simulink library "vmc"  (R2021b)
settings: Solver=VariableStepAuto  StartTime=0.0  StopTime=10.0  RelTol=1e-3
undefined symbols (not defined in the file or in its folder): AVMC_ACCDeltaTqIGain_X_kph, AVMC_ACCDeltaTqIGain_Y_mps2, AVMC_ACCDeltaTqPGain_X_kph, AVMC_ACCDeltaTqPGain_Y_kph, AVMC_ACCLongSteadyCtrl_X_kph, AVMC_AggressJerkPCT4AT_X_kph, AVMC_AggressJerkPCT_X_kph, AVMC_AggressLimitPCT4AT_X_kph, AVMC_AggressLimitPCT_X_kph, AVMC_CCLongSteadyCtrl_X_kph, AVMC_DISCDeltaTqIGain_X_kph, AVMC_DISCDeltaTqIGain_Y_mps2, AVMC_DISCDeltaTqPGain_X_kph, AVMC_DISCDeltaTqPGain_Y_kph, AVMC_DISCTrunAccJerk_X_s, AVMC_DISCTrunAccLimit_X_s, AVMC_ESCRegenOut_X_kph, AVMC_ESCRegenOut_Y_Deg, AVMC_ESCRegenOutEnSpd_X_Deg, AVMC_ISOAccLimit_X_mps, AVMC_ISODecLimit_X_mps, AVMC_ISOJerk_X_mps, AVMC_LatESCRegenOut_X_kph, AVMC_LatESCRegenOut_Y_Deg, AVMC_LongAccDeadZone_X_kph, AVMC_LongAccFiltTsforP2_X_Gps, AVMC_MCPresBaseTq_X_bar, AVMC_MSALongSteadyCtrl_X_kph, AVMC_MSAPedalOvrd2_X_kph, AVMC_MSAPedalOvrd_X_kph, AVMC_MSASpdBand_X_kph, AVMC_MSATqDownEndTq_X_kph, AVMC_MSATqDownTime_X_kph, AVMC_OPDDisSlideRate_X_Deg, AVMC_RDCDetectTime_X_kph, AVMC_RDCDetectTime_Y_pct, AVMC_RDCEnSlideRate_X_Deg, AVMC_RearWhlTqRatio_X_Nm, AVMC_RearWhlTqRatio_Y_gps, AVMC_RearWhlTqSlipGain_X_rat, AVMC_RearWhlTqSlipGain_Y_kph, AVMC_RearWhlTqSTRGGain_X_deg, AVMC_RearWhlTqSTRGGain_Y_kph, AVMC_RWSRrTSA2RWSPos_X_deg, AVMC_RWSSAS2FrtTSA_X_deg, AVMC_RWSVehSPD2RWSCoef_X_kph, AVMC_SoftJerkPCT_X_kph, AVMC_SoftLimitPCT_X_kph, AVMC_StESCYaw_X_kph, AVMC_StESCYaw_Y_Deg, AVMC_StESCYawCom_X_kph, AVMC_StESCYawCom_Y_Gps, AVMC_TMSpdBaseTq_X_rpm, AVMC_VehHoldBDecMap_X_kph, AVMC_VehHoldDecCtrlTime_X_kph, AVMC_VehHoldMCPPass_X_deg, C_TASK_10MS_S, C_TASK_5MS_S, DEG2RAD, ENUM_ACCAVAIL_AVAILABLE ... (+409)
libraries: hcu_lib x74, simulink x68, simulink_extras x3, $bdroot x2
(part 7 of 15)

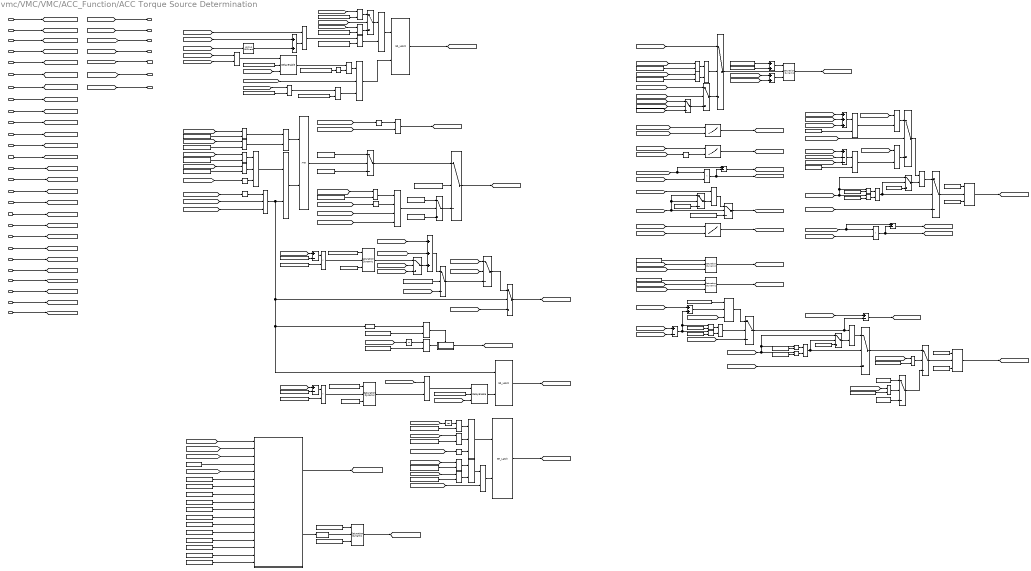
== system vmc/VMC/VMC/ACC_Function/ACC Torque Source Determination ==
  note: TRUE
  VTQD_DriverWhlTqDem_Nm : Inport
  VVMC_ADASWhlTqCal_Nm : Inport  Port=2
  VVMC_FeatArbitrFinal_enum : Inport  Port=3
  VTQD_LowIdleAccPedal_flg : Inport  Port=4
  VINP_ACCObjDist_m : Inport  Port=5
  VINP_TimeGapLevel_enum : Inport  Port=6
  VVMC_FeatArbitrSta_enum : Inport  Port=7
  VTQD_RegenMode_enum : Inport  Port=8
  VVMC_ADASActive_flg : Inport  Port=9
  task_time_s : Inport  Port=10
  VINP_LongAccel_Gps : Inport  Port=11
  VINP_VehSpeed_kph : Inport  Port=12
  VVMC_FrRrSlipSpd_kph : Inport  Port=13
  VVMC_CruzWhlTqReq_Nm : Inport  Port=14
  VVMC_CruzActive_flg : Inport  Port=15
  VVMC_MSAWhlTqReq_Nm : Inport  Port=16
  VVMC_MSAActive_flg : Inport  Port=17
  VTQD_RrEDUAvailBrkRgnTq_Nm : Inport  Port=18
  VTQD_FrEDUAvailBrkRgnTq_Nm : Inport  Port=19
  VPMM_DrivetrainSelect_enum : Inport  Port=20
  VINP_ACCObjRelSpd_mps : Inport  Port=21
  VINP_SASAngle_Deg : Inport  Port=22
  VDHP_ActAPSPosn_pct : Inport  Port=23
  VTQD_CreepBaseTqD_Nm : Inport  Port=24
  VVMC_ACCVehHoldReq_flg : Inport  Port=25
  VVMC_LongAcc_Gps : Inport  Port=26
  VVMC_ADASACCSta_enum : Inport  Port=27
  AND{,5..6,8..9,12} (6 alike) : Logic  AllPortsSameDT=off  OutDataTypeStr=boolean
  AND1 : Logic  Inputs=4  AllPortsSameDT=off  OutDataTypeStr=boolean
  AND11 : Logic  Inputs=3  AllPortsSameDT=off  OutDataTypeStr=boolean
  AND{2..4,7,13} (5 alike) : Logic  Operator=OR  AllPortsSameDT=off  OutDataTypeStr=boolean
  Abs : Abs
  Add{,9..11} (4 alike) : Sum
  Add{1,4..6,8,13} (6 alike) : Sum  Inputs=+-
  Add2 : Sum  Inputs=+++
  Add3 : Sum  Inputs=+--
  Add7 : Sum  Inputs=+++
  Cast To Single : DataTypeConversion  OutDataTypeStr=single
  Constant : Constant  Value=KVMC_ACCPedalOvrdSWC_flg
  Constant1 : Constant  Value=FALSE
  Constant10 : Constant  Value=ENUM_TIMEGAPLEVEL_LEVEL1
  Constant11 : Constant  Value=ENUM_TIMEGAPLEVEL_LEVEL2
  Constant12 : Constant  Value=ENUM_TIMEGAPLEVEL_LEVEL3
  Constant13 : Constant  Value=ENUM_TIMEGAPLEVEL_LEVEL4
  Constant14 : Constant  Value=KVMC_TimeGapBandLv2_s
  Constant15 : Constant  Value=KVMC_TimeGapBandLv3_s
  Constant16 : Constant  Value=KVMC_TimeGapBandLv4_s
  Constant17 : Constant  Value=TRUE
  Constant18 : Constant  Value=FALSE
  Constant{19,24..26,39,41..46,48,50,52,57,59,65} (17 alike) : Constant  Value=ZERO_FLOAT
  Constant2 : Constant  Value=ENUM_FEATARBITRSTA_DISC
  Constant20 : Constant  Value=FALSE
  Constant21 : Constant  Value=ENUM_FEATARBITRSTA_ACC
  Constant22 : Constant  Value=TRUE
  Constant23 : Constant  Value=KVMC_ACCPedalOvrdRestTime_s
  Constant{27..28,37,40,49,51} (6 alike) : Constant  Value=ONE_FLOAT
  Constant29 : Constant  Value=ENUM_FEATARBITRSTA_ACC
  Constant3 : Constant  Value=TRUE
  Constant30 : Constant  Value=ENUM_FEATARBITRSTA_DISC
  Constant31 : Constant  Value=KTQD_RrUppTheldTrq_Nm
  Constant32 : Constant  Value=ENUM_DRIVETRAIN_AWD  VectorParams1D=off  SampleTime=-1
  Constant33 : Constant  Value=KTQD_RrUppTheldTrq_Nm
  Constant34 : Constant  Value=KTQD_RrUppTheldTrq_Nm
  Constant35 : Constant  Value=KTQD_FrUppTheldTrq_Nm
  Constant36 : Constant  Value=KTQD_FrUppTheldTrq_Nm
  Constant38 : Constant  Value=ENUM_DRIVETRAIN_RWD  VectorParams1D=off  SampleTime=-1
  Constant4 : Constant  Value=ENUM_FEATARBITRSTA_ACC
  Constant47 : Constant  Value=KVMC_TimeGapMax_s
  Constant5 : Constant  Value=ENUM_FEATARBITRSTA_DISC
  Constant53 : Constant  Value=KVMC_ACCPedalOvrdPosn_pct
  Constant54 : Constant  Value=KVMC_ACCPedalOvrdResPosn_pct
  Constant55 : Constant  Value=KVMC_ACCOvrdMemTqSW_flg
  Constant56 : Constant  Value=KVMC_ACCOvrdTestSW_flg
  Constant58 : Constant  Value=KVMC_ACCPedalOvrdPosn4Hold_pct
  Constant6 : Constant  Value=ENUM_FEATARBITRSTA_ACCDISC
  Constant60 : Constant  Value=KVMC_ACCPedalOvrdResetSW_flg
  Constant61 : Constant  Value=KVMC_ACCPedalOvrdResetSW_flg
  Constant62 : Constant  Value=KVMC_ACCOvrdTestSW_flg
  Constant63 : Constant  Value=KVMC_ACCPedalOvrdPosn_pct
  Constant64 : Constant  Value=KVMC_ACCOvrdPedalTqRatio_Nm
  Constant66 : Constant  Value=KVMC_ACCPedalOvrdRestTime_s
  Constant67 : Constant  Value=KVMC_ACCOvrdPedalTqLinearLim_Nm
  Constant68 : Constant  Value=KVMC_ACCPedalOvrdPosn_pct
  Constant69 : Constant  Value=KVMC_ACCOvrdPedalTqRatio_Nm
  Constant7 : Constant  Value=KVMC_TimeGapMax_s
  Constant71 : Constant  Value=ENUM_ADASACCSTA_STANDBY
  Constant72 : Constant  Value=ENUM_ADASACCSTA_ACTIVE
  Constant73 : Constant  Value=ENUM_ADASACCSTA_ACTIVE
  Constant74 : Constant  Value=ENUM_ADASACCSTA_OVERRIDE
  Constant75 : Constant  Value=KVMC_ACCOvrdPedalTqLinearLim_Nm
  Constant8 : Constant  Value=KPH2MPS
  Constant9 : Constant  Value=KVMC_TimeGapBandLv1_s
  DelayEnable : hcu_lib/Basic_Blocks/DelayEnable
  DelayEnable1 : hcu_lib/Basic_Blocks/DelayEnable
  Detect Increase : simulink/Logic and Bit Operations/Detect Increase  vinit=0.0  OutDataTypeStr=boolean
  Direct Lookup Table (n-D)1 : LookupNDDirect  NumberOfTableDimensions=1  Table=MVMC_ACCPedalOvrdTqHys_Y_Nm
  Divide{,3,5,7} (4 alike) : Product  Inputs=**
  Divide1 : Product  Inputs=*/
  Divide2 : Product  Inputs=*/
  Divide4 : Product  Inputs=*/
  Equal1 : RelationalOperator  Operator===  OutDataTypeStr=boolean  RndMeth=Simplest
  Equal3 : RelationalOperator  Operator===  OutDataTypeStr=boolean  RndMeth=Simplest
  Logical Operator : Logic  Operator=OR  AllPortsSameDT=off  OutDataTypeStr=boolean
  Logical Operator1 : Logic  Inputs=3  AllPortsSameDT=off  OutDataTypeStr=boolean
  Logical Operator2 : Logic  Operator=OR  AllPortsSameDT=off  OutDataTypeStr=boolean
  Logical Operator3 : Logic  Inputs=3  AllPortsSameDT=off  OutDataTypeStr=boolean
  Logical Operator4 : Logic  AllPortsSameDT=off  OutDataTypeStr=boolean
  Logical Operator5 : Logic  Operator=OR  AllPortsSameDT=off  OutDataTypeStr=boolean
  MMAP_RearWhlTqSlipGain_Z_Nm : Lookup_n-D  BreakpointsForDimension1=AVMC_RearWhlTqSlipGain_Y_kph  BreakpointsForDimension2=AVMC_RearWhlTqSlipGain_X_rat  Table=MVMC_RearWhlTqSlipGain_Z_Nm  InternalRulePriority=Speed  RndMeth=Simplest  InputSameDT=on
      settings: InputPortMap=u0,u1
  MVMC_RearWhlTqRatio_Z_rat : Lookup_n-D  BreakpointsForDimension1=AVMC_RearWhlTqRatio_Y_gps  BreakpointsForDimension2=AVMC_RearWhlTqRatio_X_Nm  Table=MVMC_RearWhlTqRatio_Z_rat  InternalRulePriority=Speed  RndMeth=Simplest  InputSameDT=on
      settings: InputPortMap=u0,u1
  MVMC_RearWhlTqSTRGGain_Z_Nm : Lookup_n-D  BreakpointsForDimension1=AVMC_RearWhlTqSTRGGain_Y_kph  BreakpointsForDimension2=AVMC_RearWhlTqSTRGGain_X_deg  Table=MVMC_RearWhlTqSTRGGain_Z_Nm  InternalRulePriority=Speed  RndMeth=Simplest  InputSameDT=on
      settings: InputPortMap=u0,u1
  Max : MinMax  Function=max  Inputs=2
  Max1 : MinMax  Inputs=2
  Max2 : MinMax  Inputs=2
  Max3 : MinMax  Function=max  Inputs=2
  Min : MinMax  Function=max  Inputs=2
  NOT{,1..5} (6 alike) : Logic  Operator=NOT  AllPortsSameDT=off  OutDataTypeStr=boolean
  OR1 : Logic  Operator=OR  Inputs=3  AllPortsSameDT=off  OutDataTypeStr=boolean
  Relational Operator{,7,11,13,19} (5 alike) : RelationalOperator  Operator=>  OutDataTypeStr=boolean  RndMeth=Simplest
  Relational Operator{1..6,9,21..22} (9 alike) : RelationalOperator  Operator===  OutDataTypeStr=boolean  RndMeth=Simplest
  Relational Operator{10,12,14,16} (4 alike) : RelationalOperator  Operator=<  OutDataTypeStr=boolean  RndMeth=Simplest
  Relational Operator15 : RelationalOperator  OutDataTypeStr=boolean  RndMeth=Simplest
  Relational Operator17 : RelationalOperator  OutDataTypeStr=boolean  RndMeth=Simplest
  Relational Operator23 : RelationalOperator  Operator=~=  OutDataTypeStr=boolean  RndMeth=Simplest
  Relational Operator24 : RelationalOperator  Operator=~=  OutDataTypeStr=boolean  RndMeth=Simplest
  Relational Operator8 : RelationalOperator  Operator=<=  OutDataTypeStr=boolean  RndMeth=Simplest
  SR_Latch : hcu_lib/Basic_Blocks/SR_Latch
  SR_Latch1 : hcu_lib/Basic_Blocks/SR_Latch
  SR_Latch2 : hcu_lib/Basic_Blocks/SR_Latch
  Saturation Dynamic{,1..8} (9 alike) : simulink/Discontinuities/Saturation Dynamic  OutMin=[]  OutMax=[]  OutDataTypeStr=Inherit: Same as second input  OutDataType=fixdt(1, 16)  OutScaling=2^-10  DoSatur=off
  Switch{,4..7,9..10,12,15} (9 alike) : Switch  Criteria=u2 > Threshold
  Switch{1,3,8,11,13} (5 alike) : Switch  Criteria=u2 ~= 0
  Switch2 : Switch
  TimeGapJudgement : Stateflow chart  TreatAsAtomicUnit=on
  Triggered Subsystem2 : Subsystem  TreatAsAtomicUnit=on
  Unit Delay : UnitDelay  SampleTime=-1  HasFrameUpgradeWarning=on
  Unit Delay1 : UnitDelay  SampleTime=-1  HasFrameUpgradeWarning=on
  u2 > 0 : Switch  Criteria=u2 > Threshold
  u2 > 0 (1) : Switch  Criteria=u2 > Threshold
  u2 > 0 (1)1 : Switch  Criteria=u2 > Threshold
  u2 > 0 (1)2 : Switch  Criteria=u2 > Threshold
  u2 > 0 (2) : Switch  Criteria=u2 > Threshold
  u2 > 0 (3) : Switch  Criteria=u2 > Threshold
  VVMC_ACCPedalOvrd_flg : Outport
  VVMC_ADASWhlTqReq_Nm : Outport  Port=2
  VVMC_TimeGapCalcu_s : Outport  Port=3
  VVMC_AccPedalOvrdDISC_flg : Outport  Port=4
  VVMC_RearTqRatio_rat : Outport  Port=5
  VVMC_TimeGapJudge_flag : Outport  Port=6
  VVMC_ACCOvrdMemTq_Nm : Outport  Port=7
  wires:
  [VVMC_ACCPedalTqEnOvrd_flg] -> Logical Operator1/2
  [VVMC_ADASActive_flg] -> AND1/4
  [VVMC_ACCPedalTqEnOvrd_flg] -> AND1/3
  [VVMC_ADASWhlTqCal_Nm] -> Relational Operator8/2
  [VTQD_DriverWhlTqDem_Nm] -> Relational Operator7/1
  Relational Operator8/1 -> DelayEnable/1
  SR_Latch/1 -> [VVMC_ACCPedalTqEnOvrd_flg]  "VVMC_ACCPedalTqEnOvrd_flg"
  Direct Lookup Table (n-D)1/1 -> Add/2  "VVMC_ACCPedalOvrdTqHys_Nm"
  [VTQD_DriverWhlTqDem_Nm] -> Relational Operator8/1
  Relational Operator7/1 -> AND7/1
  Add/1 -> Relational Operator7/2
  [VVMC_ADASWhlTqCal_Nm] -> Add/1
  [VTQD_RegenMode_enum] -> Direct Lookup Table (n-D)1/1
  VVMC_ADASActive_flg/1 -> [VVMC_ADASActive_flg]
  VTQD_RegenMode_enum/1 -> [VTQD_RegenMode_enum]
  Saturation Dynamic2/1 -> [VVMC_TimeGapCalcu_s]  "VVMC_TimeGapCalcu_s"
  Constant/1 -> u2 > 0 (3)/2
  u2 > 0/1 -> u2 > 0 (3)/1
  u2 > 0 (2)/1 -> u2 > 0 (3)/3
  [VVMC_FeatArbitrFinal_enum] -> Relational Operator6/1
  Constant21/1 -> Relational Operator6/2
  Constant22/1 -> u2 > 0 (2)/1
  Constant20/1 -> u2 > 0 (2)/3
  NOT2/1 -> AND1/2
  [VTQD_LowIdleAccPedal_flg] -> NOT2/1
  AND1/1 -> u2 > 0 (2)/2
  Relational Operator6/1 -> AND1/1
  [VVMC_TimeGapCalcu_s] -> VVMC_TimeGapCalcu_s/1
  TimeGapJudgement/2(VVMC_TimeGapCalcu_s) -> Cast To Single/1
  Constant7/1 -> TimeGapJudgement/17(KVMC_TimeGapMax_s)
  Constant6/1 -> Relational Operator4/2
  [VVMC_FeatArbitrSta_enum] -> Relational Operator4/1
  Relational Operator4/1 -> Logical Operator3/1
  VVMC_FeatArbitrSta_enum/1 -> [VVMC_FeatArbitrSta_enum]
  Constant19/1 -> TimeGapJudgement/16(ZERO_FLOAT)
  Constant18/1 -> TimeGapJudgement/15(FALSE)
  Constant17/1 -> TimeGapJudgement/14(TRUE)
  Constant16/1 -> TimeGapJudgement/13(KVMC_TimeGapBandLv4_s)
  Constant13/1 -> TimeGapJudgement/12(ENUM_TIMEGAPLEVEL_LEVEL4)
  Constant15/1 -> TimeGapJudgement/11(KVMC_TimeGapBandLv3_s)
  Constant12/1 -> TimeGapJudgement/10(ENUM_TIMEGAPLEVEL_LEVEL3)
  Constant14/1 -> TimeGapJudgement/9(KVMC_TimeGapBandLv2_s)
  Constant11/1 -> TimeGapJudgement/8(ENUM_TIMEGAPLEVEL_LEVEL2)
  Constant9/1 -> TimeGapJudgement/7(KVMC_TimeGapBandLv1_s)
  Constant10/1 -> TimeGapJudgement/6(ENUM_TIMEGAPLEVEL_LEVEL1)
  [VVMC_TimeGapJudge_flag] -> NOT1/1
  NOT1/1 -> Logical Operator3/3
  Relational Operator1/1 -> Logical Operator3/2
  TimeGapJudgement/1(VVMC_TimeGapJudge_flag) -> [VVMC_TimeGapJudge_flag]  "VVMC_TimeGapJudge_flag"
  [VINP_ACCObjDist_m] -> TimeGapJudgement/2(VINP_ACCObjDist_m)
  [VINP_VehSpeed_kph] -> TimeGapJudgement/3(VINP_VehSpeed_kph)
  Constant8/1 -> TimeGapJudgement/4(KPH2MPS)
  [VINP_TimeGapLevel_enum] -> TimeGapJudgement/5(VINP_TimeGapLevel_enum)
  VINP_TimeGapLevel_enum/1 -> [VINP_TimeGapLevel_enum]
  VINP_ACCObjDist_m/1 -> [VINP_ACCObjDist_m]
  Logical Operator2/1 -> AND/1
  Relational Operator3/1 -> Logical Operator2/2
  Constant5/1 -> Relational Operator3/2
  [VVMC_FeatArbitrFinal_enum] -> Relational Operator3/1
  Logical Operator/1 -> AND/2
  Logical Operator3/1 -> Logical Operator/1
  [VVMC_FeatArbitrFinal_enum] -> Relational Operator1/1
  Constant2/1 -> Relational Operator1/2
  Constant4/1 -> Relational Operator2/2
  [VVMC_FeatArbitrFinal_enum] -> Relational Operator2/1
  VTQD_DriverWhlTqDem_Nm/1 -> [VTQD_DriverWhlTqDem_Nm]
  VVMC_ADASWhlTqCal_Nm/1 -> [VVMC_ADASWhlTqCal_Nm]
  [VVMC_ACCPedalOvrd_flg] -> VVMC_ACCPedalOvrd_flg/1
  [VVMC_ADASWhlTqReq_Nm] -> VVMC_ADASWhlTqReq_Nm/1
  u2 > 0 (1)/1 -> [VVMC_ADASWhlTqReq_Nm]  "VVMC_ADASWhlTqReq_Nm"
  [VVMC_ADASWhlTqCal_Nm] -> u2 > 0 (1)/3
  Constant1/1 -> u2 > 0/3
  Constant3/1 -> u2 > 0/1
  u2 > 0 (3)/1 -> [VVMC_ACCPedalOvrd_flg]  "VVMC_ACCPedalOvrd_flg"
  AND/1 -> u2 > 0/2
  Relational Operator2/1 -> Logical Operator2/1
  VVMC_FeatArbitrFinal_enum/1 -> [VVMC_FeatArbitrFinal_enum]
  VTQD_LowIdleAccPedal_flg/1 -> [VTQD_LowIdleAccPedal_flg]
  NOT/1 -> Logical Operator1/1
  [VTQD_LowIdleAccPedal_flg] -> NOT/1
  [VVMC_AccPedalOvrdDISC_flg] -> VVMC_AccPedalOvrdDISC_flg/1
  Logical Operator4/1 -> [VVMC_AccPedalOvrdDISC_flg]  "VVMC_AccPedalOvrdDISC_flg"
  NOT3/1 -> Logical Operator4/1
  [VVMC_ACCPedalTqEnOvrd_flg] -> Logical Operator4/2
  [VTQD_LowIdleAccPedal_flg] -> NOT3/1
  [task_time_s] -> DelayEnable/3
  DelayEnable/1 -> AND9/1
  Constant23/1 -> DelayEnable/2
  [VTQD_LowIdleAccPedal_flg] -> OR1/2
  OR1/1 -> SR_Latch/2
  task_time_s/1 -> [task_time_s]
  [VVMC_VMCWhlTq4RatioCalcu_Nm] -> MVMC_RearWhlTqRatio_Z_rat/2
  VINP_LongAccel_Gps/1 -> [VINP_LongAccel_Gps]
  [VINP_LongAccel_Gps] -> MVMC_RearWhlTqRatio_Z_rat/1
  MVMC_RearWhlTqRatio_Z_rat/1 -> [VVMC_RearTqRatioBfrSlip_rat]  "VVMC_RearTqRatioBfrSlip_rat"
  [VVMC_RearTqRatio_rat] -> VVMC_RearTqRatio_rat/1
  VINP_VehSpeed_kph/1 -> [VINP_VehSpeed_kph]
  VVMC_FrRrSlipSpd_kph/1 -> [VVMC_FrRrSlipSpd_kph]
  [VVMC_VMCWhlTq4RatioCalcu_Nm] -> Divide/1, Add1/1
  [VVMC_RearTqRatioBfrSlip_rat] -> Divide/2
  Divide/1 -> [VVMC_ADASRrWhlTqBfrSlip_Nm], Add1/2  "VVMC_ADASRrWhlTqBfrSlip_Nm"
  Add1/1 -> [VVMC_ADASFrWhlTqBfrSlip_Nm]  "VVMC_ADASFrWhlTqBfrSlip_Nm"
  [VINP_VehSpeed_kph] -> Switch/2, Switch4/2, Switch4/1
  Constant24/1 -> Switch/3
  Divide1/1 -> Switch/1
  [VVMC_FrRrSlipSpd_kph] -> Divide1/1
  Switch/1 -> [VVMC_FrRrSlipRate_rat]  "VVMC_FrRrSlipRate_rat"
  [VVMC_FrRrSlipRate_rat] -> MMAP_RearWhlTqSlipGain_Z_Nm/2
  [VINP_VehSpeed_kph] -> MMAP_RearWhlTqSlipGain_Z_Nm/1
  MMAP_RearWhlTqSlipGain_Z_Nm/1 -> [VVMC_RearWhlTqSlipGain_Nm]  "VVMC_RearWhlTqSlipGain_Nm"
  [VVMC_RearTqRatioBfrSlip_rat] -> Switch1/3
  Saturation Dynamic5/1 -> [VVMC_RearTqRatioAftSlip_rat]  "VVMC_RearTqRatioAftSlip_rat"
  Switch2/1 -> Divide2/1
  Divide2/1 -> Switch1/1
  Constant27/1 -> Switch3/3
  Switch3/1 -> Divide2/2
  Constant28/1 -> Switch4/3
  Switch4/1 -> Divide1/2
  [VVMC_ADASActive_flg] -> Logical Operator1/3
  Relational Operator5/1 -> Logical Operator5/1
  Relational Operator9/1 -> Logical Operator5/2
  [VVMC_FeatArbitrFinal_enum] -> Relational Operator5/1
  Constant30/1 -> Relational Operator9/2
  [VVMC_FeatArbitrFinal_enum] -> Relational Operator9/1
  Constant29/1 -> Relational Operator5/2
  Logical Operator5/1 -> Switch5/2
  [VTQD_DriverWhlTqDem_Nm] -> Switch7/3
  [VVMC_ADASWhlTqReq_Nm] -> Switch5/1
  Saturation Dynamic4/1 -> [VVMC_VMCWhlTq4RatioCalcu_Nm]  "VVMC_VMCWhlTq4RatioCalcu_Nm"
  VVMC_MSAActive_flg/1 -> [VVMC_MSAActive_flg]
  VVMC_MSAWhlTqReq_Nm/1 -> [VVMC_MSAWhlTqReq_Nm]
  VVMC_CruzWhlTqReq_Nm/1 -> [VVMC_CruzWhlTqReq_Nm]
  VVMC_CruzActive_flg/1 -> [VVMC_CruzActive_flg]
  [VVMC_CruzActive_flg] -> Switch6/2
  [VVMC_CruzWhlTqReq_Nm] -> Switch6/1
  Switch6/1 -> Switch5/3
  [VVMC_MSAActive_flg] -> Switch7/2
  [VVMC_MSAWhlTqReq_Nm] -> Switch7/1
  Switch7/1 -> Switch6/3
  Add4/1 -> [VVMC_ADASFrWhlTqAftSlip_Nm]  "VVMC_ADASFrWhlTqAftSlip_Nm"
  Divide3/1 -> Add4/2, [VVMC_ADASRrWhlTqAftSlip_Nm]  "VVMC_ADASRrWhlTqAftSlip_Nm"
  [VVMC_RearTqRatioAftSlip_rat] -> Divide3/2
  [VVMC_VMCWhlTq4RatioCalcu_Nm] -> Add4/1, Divide3/1
  VTQD_FrEDUAvailBrkRgnTq_Nm/1 -> [VTQD_FrEDUAvailBrkRgnTq_Nm]
  VTQD_RrEDUAvailBrkRgnTq_Nm/1 -> [VTQD_RrEDUAvailBrkRgnTq_Nm]
  [VVMC_ADASFrWhlTqAftSlip_Nm] -> Saturation Dynamic/2
  Constant35/1 -> Saturation Dynamic/1
  [VTQD_FrEDUAvailBrkRgnTq_Nm] -> Saturation Dynamic/3
  Constant31/1 -> Saturation Dynamic1/1
  [VVMC_ADASRrWhlTqAftSlip_Nm] -> Saturation Dynamic1/2
  [VTQD_RrEDUAvailBrkRgnTq_Nm] -> Saturation Dynamic1/3
  Saturation Dynamic/1 -> [VVMC_ADASFrWhlTqAftLim_Nm]  "VVMC_ADASFrWhlTqAftLim_Nm"
  Saturation Dynamic1/1 -> [VVMC_ADASRrWhlTqAftLim_Nm]  "VVMC_ADASRrWhlTqAftLim_Nm"
  [VVMC_ADASFrWhlTqAftSlip_Nm] -> Add5/1
  [VVMC_ADASFrWhlTqAftLim_Nm] -> Add5/2
  [VVMC_ADASRrWhlTqAftLim_Nm] -> Switch8/3
  Saturation Dynamic3/1 -> Switch8/1
  [VVMC_ADASRrWhlTqAftLim_Nm] -> Add9/1
  Constant33/1 -> Saturation Dynamic3/1
  [VTQD_RrEDUAvailBrkRgnTq_Nm] -> Saturation Dynamic3/3
  Add9/1 -> Saturation Dynamic3/2
  Switch13/1 -> Divide4/2
  Constant37/1 -> Switch13/3
  Divide4/1 -> Switch11/1
  Switch8/1 -> Add6/2, Divide4/1  "VVMC_ADASRrWhlTq_Nm"
  Saturation Dynamic6/1 -> [VVMC_RearTqRatio_rat]  "VVMC_RearTqRatio_rat"
  [VVMC_RearTqRatioBfrSlip_rat] -> Switch11/3
  [VTQD_RrEDUAvailBrkRgnTq_Nm] -> Add11/2
  Constant34/1 -> Add10/2
  [VTQD_FrEDUAvailBrkRgnTq_Nm] -> Add11/1
  Constant36/1 -> Add10/1
  Add10/1 -> Saturation Dynamic4/1
  Add11/1 -> Saturation Dynamic4/3
  Switch5/1 -> Saturation Dynamic4/2
  [VVMC_VMCWhlTq4RatioCalcu_Nm] -> Add6/1
  Add6/1 -> [VVMC_ADASFrWhlTq_Nm]  "VVMC_ADASFrWhlTq_Nm"
  VPMM_DrivetrainSelect_enum/1 -> [VPMM_DrivetrainSelect_enum]
  [VPMM_DrivetrainSelect_enum] -> Equal3/1
  Constant32/1 -> Equal3/2
  Switch11/1 -> Switch9/1
  Equal3/1 -> Switch9/2
  Constant38/1 -> Equal1/2
  [VPMM_DrivetrainSelect_enum] -> Equal1/1
  Equal1/1 -> Switch10/2
  Switch10/1 -> Switch9/3
  Constant39/1 -> Switch10/3
  Constant40/1 -> Switch10/1
  Constant42/1 -> Relational Operator10/2
  Relational Operator/1 -> AND2/1
  Relational Operator10/1 -> AND2/2
  Constant41/1 -> Relational Operator/2
  [VVMC_VMCWhlTq4RatioCalcu_Nm] -> Relational Operator10/1, Switch3/1, Relational Operator/1
  AND2/1 -> Switch3/2, Switch1/2
  Constant44/1 -> Relational Operator12/2
  Relational Operator11/1 -> AND3/1
  Relational Operator12/1 -> AND3/2
  Constant43/1 -> Relational Operator11/2
  Add5/1 -> Relational Operator11/1, Add9/2, Relational Operator12/1
  AND3/1 -> Switch8/2
  Constant46/1 -> Relational Operator14/2
  Relational Operator13/1 -> AND4/1
  Relational Operator14/1 -> AND4/2
  Constant45/1 -> Relational Operator13/2
  [VVMC_VMCWhlTq4RatioCalcu_Nm] -> Relational Operator14/1, Switch13/1, Relational Operator13/1
  AND4/1 -> Switch13/2, Switch11/2
  VINP_ACCObjRelSpd_mps/1 -> [VINP_ACCObjRelSpd_mps]
  [VINP_ACCObjRelSpd_mps] -> TimeGapJudgement/1(VINP_ACCObjRelSpd_mps)
  Cast To Single/1 -> Saturation Dynamic2/2
  Constant47/1 -> Saturation Dynamic2/1
  Constant48/1 -> Saturation Dynamic2/3
  [VVMC_TimeGapJudge_flag] -> VVMC_TimeGapJudge_flag/1
  Abs/1 -> MVMC_RearWhlTqSTRGGain_Z_Nm/2
  [VINP_VehSpeed_kph] -> MVMC_RearWhlTqSTRGGain_Z_Nm/1
  [VINP_SASAngle_Deg] -> Abs/1
  MVMC_RearWhlTqSTRGGain_Z_Nm/1 -> [VVMC_RearWhlTqSTRGGain_Nm]  "VVMC_RearWhlTqSTRGGain_Nm"
  [VVMC_RearWhlTqSTRGGain_Nm] -> Add2/3
  [VVMC_RearWhlTqSTRGGain_Nm] -> Add3/3
  [VVMC_ADASRrWhlTqBfrSlip_Nm] -> Add2/1
  [VVMC_RearWhlTqSlipGain_Nm] -> Add3/2
  Max1/1 -> Max3/2
  Add2/1 -> Max/1
  [VVMC_VMCWhlTq4RatioCalcu_Nm] -> Switch2/2
  [VVMC_RearWhlTqSlipGain_Nm] -> Add2/2
  Constant25/1 -> Max/2
  Add3/1 -> Max1/1
  Constant26/1 -> Max1/2
  [VVMC_ADASRrWhlTqBfrSlip_Nm] -> Add3/1
  Max/1 -> Max2/2
  VINP_SASAngle_Deg/1 -> [VINP_SASAngle_Deg]
  [VVMC_VMCWhlTq4RatioCalcu_Nm] -> Max2/1
  Max2/1 -> Switch2/1
  [VVMC_VMCWhlTq4RatioCalcu_Nm] -> Max3/1
  Max3/1 -> Switch2/3
  Constant49/1 -> Saturation Dynamic5/1
  Switch1/1 -> Saturation Dynamic5/2
  Constant50/1 -> Saturation Dynamic5/3
  Constant52/1 -> Saturation Dynamic6/3
  Switch9/1 -> Saturation Dynamic6/2
  Constant51/1 -> Saturation Dynamic6/1
  [VDHP_ActAPSPosn_pct] -> Relational Operator15/1
  Relational Operator15/1 -> Switch12/3
  AND5/1 -> SR_Latch/1
  Constant53/1 -> Relational Operator15/2
  VDHP_ActAPSPosn_pct/1 -> [VDHP_ActAPSPosn_pct]
  VTQD_CreepBaseTqD_Nm/1 -> [VTQD_CreepBaseTqD_Nm]
  [VTQD_CreepBaseTqD_Nm] -> Add7/2
  Switch15/1 -> Add7/3
  Triggered Subsystem2/1(Out1) -> [VVMC_ACCOvrdMemTq_Nm]  "VVMC_ACCOvrdMemTq_Nm"
  Detect Increase/1 -> AND6/1
  Unit Delay/1 -> Min/1
  Logical Operator1/1 -> SR_Latch1/1, Detect Increase/1, u2 > 0 (1)/2, Logical Operator/2
  [VVMC_ADASWhlTqReq_Nm] -> Unit Delay/1
  Add7/1 -> u2 > 0 (1)1/1
  [VVMC_ACCOvrdMemTq_Nm] -> Add7/1
  Constant55/1 -> AND6/2
  AND6/1 -> Triggered Subsystem2/Trigger
  AND7/1 -> AND5/2
  Constant56/1 -> AND7/2
  Min/1 -> Triggered Subsystem2/1(In1)
  Constant57/1 -> Min/2
  [VVMC_ACCOvrdMemTq_Nm] -> VVMC_ACCOvrdMemTq_Nm/1
  VVMC_ACCVehHoldReq_flg/1 -> [VVMC_ACCVehHoldReq_flg]
  [VVMC_ACCVehHoldReq_flg] -> Switch12/2
  Switch12/1 -> AND5/1
  Constant58/1 -> Relational Operator17/2
  [VDHP_ActAPSPosn_pct] -> Relational Operator17/1
  Relational Operator17/1 -> Switch12/1
  AND8/1 -> OR1/3
  Constant60/1 -> AND8/2
  Constant61/1 -> NOT4/1
  AND9/1 -> OR1/1
  NOT4/1 -> AND9/2
  [VDHP_ActAPSPosn_pct] -> Add8/1
  Constant63/1 -> Add8/2
  Add8/1 -> Divide5/1
  Constant64/1 -> Divide5/2
  [VTQD_DriverWhlTqDem_Nm] -> Relational Operator19/1
  Saturation Dynamic8/1 -> Relational Operator19/2
  Relational Operator19/1 -> DelayEnable1/1
  SR_Latch1/1 -> [VVMC_ACCOvrdBackDrTq_flg]  "VVMC_ACCOvrdBackDrTq_flg"
  [VVMC_ACCOvrdBackDrTq_flg] -> Switch15/2
  Divide5/1 -> Saturation Dynamic7/2
  [VTQD_DriverWhlTqDem_Nm] -> Switch15/3
  Constant66/1 -> DelayEnable1/2
  [task_time_s] -> DelayEnable1/3
  DelayEnable1/1 -> SR_Latch1/2
  Saturation Dynamic7/1 -> Switch15/1
  Constant69/1 -> Divide7/2
  Add13/1 -> Divide7/1
  Constant68/1 -> Add13/2
  [VDHP_ActAPSPosn_pct] -> Add13/1
  Constant62/1 -> u2 > 0 (1)1/2
  [VTQD_DriverWhlTqDem_Nm] -> u2 > 0 (1)1/3
  u2 > 0 (1)1/1 -> u2 > 0 (1)2/3
  VVMC_LongAcc_Gps/1 -> [VVMC_LongAcc_Gps]
  Relational Operator16/1 -> AND8/1
  VVMC_ADASACCSta_enum/1 -> [VVMC_ADASACCSta_enum]
  [VVMC_ADASACCSta_enum] -> Unit Delay1/1
  Unit Delay1/1 -> Relational Operator21/1
  Constant71/1 -> Relational Operator21/2
  Constant72/1 -> Relational Operator22/2
  [VVMC_ADASACCSta_enum] -> Relational Operator22/1
  [VTQD_LowIdleAccPedal_flg] -> NOT5/1
  Relational Operator22/1 -> AND11/2
  Relational Operator21/1 -> AND11/1
  NOT5/1 -> AND11/3
  AND11/1 -> SR_Latch2/1
  SR_Latch2/1 -> [VVMC_ACCActivePedalOn_flg]  "VVMC_ACCActivePedalOn_flg"
  [VTQD_LowIdleAccPedal_flg] -> AND13/2
  [VVMC_ADASACCSta_enum] -> Relational Operator23/1
  Constant73/1 -> Relational Operator23/2
  Constant74/1 -> Relational Operator24/2
  [VVMC_ADASACCSta_enum] -> Relational Operator24/1
  Relational Operator23/1 -> AND12/1
  Relational Operator24/1 -> AND12/2
  AND12/1 -> AND13/1
  AND13/1 -> SR_Latch2/2
  [VVMC_ACCActivePedalOn_flg] -> u2 > 0 (1)2/2
  [VTQD_DriverWhlTqDem_Nm] -> u2 > 0 (1)2/1
  u2 > 0 (1)2/1 -> u2 > 0 (1)/1
  [VDHP_ActAPSPosn_pct] -> Relational Operator16/1
  Constant54/1 -> Relational Operator16/2
  Constant59/1 -> Saturation Dynamic7/3
  Constant75/1 -> Saturation Dynamic7/1
  Constant67/1 -> Saturation Dynamic8/1
  Constant65/1 -> Saturation Dynamic8/3
  Divide7/1 -> Saturation Dynamic8/2

== system vmc/VMC/VMC/ACC_Function/Hand Shaking ==
  VVMC_FeatArbitrFinal_enum : Inport
  VVMC_ACCCtrlAllow_flg : Inport  Port=2
  Constant1 : Constant  Value=TRUE
  Constant2 : Constant  Value=ENUM_FEATARBITRSTA_DISC
  Constant3 : Constant  Value=FALSE
  Constant4 : Constant  Value=ENUM_FEATARBITRSTA_ACC
  Constant5 : Constant  Value=TRUE
  Constant6 : Constant  Value=FALSE
  Logical Operator : Logic  AllPortsSameDT=off  OutDataTypeStr=boolean
  Logical Operator1 : Logic  Operator=OR  AllPortsSameDT=off  OutDataTypeStr=boolean
  Relational Operator1 : RelationalOperator  Operator===  OutDataTypeStr=boolean  RndMeth=Simplest
  Relational Operator2 : RelationalOperator  Operator===  OutDataTypeStr=boolean  RndMeth=Simplest
  Switch : Switch  Criteria=u2 > Threshold
  u2>0 : Switch  Criteria=u2 > Threshold
  VVMC_ACCCtrlAvail_flg : Outport
  VVMC_ADASActive_flg : Outport  Port=2
  wires:
  Logical Operator1/1 -> Logical Operator/1
  Relational Operator2/1 -> Logical Operator1/1
  Constant4/1 -> Relational Operator2/2
  [VVMC_FeatArbitrFinal_enum] -> Relational Operator2/1
  [VVMC_ACCCtrlAvail_flg] -> VVMC_ACCCtrlAvail_flg/1
  VVMC_FeatArbitrFinal_enum/1 -> [VVMC_FeatArbitrFinal_enum]
  [VVMC_FeatArbitrFinal_enum] -> Relational Operator1/1
  Constant2/1 -> Relational Operator1/2
  [VVMC_ADASActive_flg] -> VVMC_ADASActive_flg/1
  [VVMC_ACCCtrlAllow_flg] -> Logical Operator/2, Switch/2
  Switch/1 -> [VVMC_ACCCtrlAvail_flg]  "VVMC_ACCCtrlAvail_flg"
  Constant6/1 -> Switch/3
  Constant5/1 -> Switch/1
  VVMC_ACCCtrlAllow_flg/1 -> [VVMC_ACCCtrlAllow_flg]
  Relational Operator1/1 -> Logical Operator1/2
  Logical Operator/1 -> u2>0/2
  Constant1/1 -> u2>0/1
  u2>0/1 -> [VVMC_ADASActive_flg]  "VVMC_ADASActive_flg"
  Constant3/1 -> u2>0/3

== system vmc/VMC/VMC/APS function/CAAS HandShake ==
  VINP_VehSpeed_kph : Inport
  VVMC_ADASActive_flg : Inport  Port=2
  VVMC_CruzActive_flg : Inport  Port=3
  task_time_s : Inport  Port=4
  VINP_CAASVMCReqA_flg : Inport  Port=5
  AND : Logic  Inputs=3  AllPortsSameDT=off  OutDataTypeStr=boolean
  AND1 : Logic  AllPortsSameDT=off  OutDataTypeStr=boolean
  Constant1 : Constant  Value=KVMC_CAASCtrlAllowTime_s
  Constant11 : Constant  Value=KVMC_CAASEnVehSpd_kph
  Constant2 : Constant  Value=KVMC_CAASVMCReqA_flg_ovrdflg
  Constant3 : Constant  Value=KVMC_CAASVMCReqA_flg_ovrdval
  DelayEnable : hcu_lib/Basic_Blocks/DelayEnable
  NOT : Logic  Operator=NOT  AllPortsSameDT=off  OutDataTypeStr=boolean
  NOT1 : Logic  Operator=NOT  AllPortsSameDT=off  OutDataTypeStr=boolean
  Relational Operator : RelationalOperator  Operator=<=  OutDataTypeStr=boolean  RndMeth=Simplest
  Switch : Switch  Criteria=u2 > Threshold
  VVMC_CAASCtrlAvail_flg : Outport
  VVMC_CAASActive_flg : Outport  Port=2
  wires:
  Relational Operator/1 -> AND/1
  VVMC_ADASActive_flg/1 -> [VVMC_ADASActive_flg]
  VINP_VehSpeed_kph/1 -> [VINP_VehSpeed_kph]
  AND/1 -> DelayEnable/1
  Constant1/1 -> DelayEnable/2
  task_time_s/1 -> [task_time_s]
  [VINP_VehSpeed_kph] -> Relational Operator/1
  [VVMC_CruzActive_flg] -> NOT1/1
  VVMC_CruzActive_flg/1 -> [VVMC_CruzActive_flg]
  Constant11/1 -> Relational Operator/2
  DelayEnable/1 -> [VVMC_CAASCtrlAvail_flg]  "VVMC_CAASCtrlAvail_flg"
  [task_time_s] -> DelayEnable/3
  NOT1/1 -> AND/3
  NOT/1 -> AND/2
  [VVMC_ADASActive_flg] -> NOT/1
  [VVMC_CAASCtrlAvail_flg] -> VVMC_CAASCtrlAvail_flg/1
  [VVMC_CAASCtrlAvail_flg] -> AND1/1
  VINP_CAASVMCReqA_flg/1 -> [VINP_CAASVMCReqA_flg]
  AND1/1 -> [VVMC_CAASActive_flg]  "VVMC_CAASActive_flg"
  [VVMC_CAASActive_flg] -> VVMC_CAASActive_flg/1
  [VINP_CAASVMCReqA_flg] -> Switch/3
  Switch/1 -> AND1/2
  Constant3/1 -> Switch/1
  Constant2/1 -> Switch/2

== system vmc/VMC/VMC/APS function/Command Determination1 ==
  VVMC_APSActive_flg : Inport
  VINP_APSStaSys_enum : Inport  Port=2
  VINP_APSShiftPosnReq_enum : Inport  Port=3
  VINP_APSSpeedCMD_kph : Inport  Port=4
  AND : Logic  AllPortsSameDT=off  OutDataTypeStr=boolean
  Constant : Constant  Value=ENUM_APSSYSTEMSTA_ACTIVE
  Constant1 : Constant  Value=ENUM_APSSYSTEMSTA_REMOTEACTIVE
  Constant2 : Constant  Value=ZERO_FLOAT
  Constant3 : Constant  Value=ENUM_APSSHIFTPOSNREQ_PARK
  Equal : RelationalOperator  Operator===  OutDataTypeStr=boolean  RndMeth=Simplest
  Equal1 : RelationalOperator  Operator===  OutDataTypeStr=boolean  RndMeth=Simplest
  OR : Logic  Operator=OR  AllPortsSameDT=off  OutDataTypeStr=boolean
  Switch : Switch  Criteria=u2 > Threshold
  Switch1 : Switch  Criteria=u2 > Threshold
  VVMC_APSSpeedCMD_kph : Outport
  VVMC_APSShiftPosnReq_enum : Outport  Port=2
  wires:
  [VVMC_APSEnCMD_flg] -> Switch1/2
  [VINP_APSShiftPosnReq_enum] -> Switch1/1
  Constant3/1 -> Switch1/3
  Switch1/1 -> VVMC_APSShiftPosnReq_enum/1  "VVMC_APSShiftPosnReq_enum"
  Switch/1 -> VVMC_APSSpeedCMD_kph/1  "VVMC_APSSpeedCMD_kph"
  Constant2/1 -> Switch/3
  [VINP_APSSpeedCMD_kph] -> Switch/1
  [VVMC_APSEnCMD_flg] -> Switch/2
  AND/1 -> [VVMC_APSEnCMD_flg]  "VVMC_APSEnCMD_flg"
  OR/1 -> AND/2
  [VVMC_APSActive_flg] -> AND/1
  Equal1/1 -> OR/2
  Equal/1 -> OR/1
  [VINP_APSStaSys_enum] -> Equal1/1
  Constant1/1 -> Equal1/2
  Constant/1 -> Equal/2
  [VINP_APSStaSys_enum] -> Equal/1
  VINP_APSSpeedCMD_kph/1 -> [VINP_APSSpeedCMD_kph]
  VINP_APSShiftPosnReq_enum/1 -> [VINP_APSShiftPosnReq_enum]
  VINP_APSStaSys_enum/1 -> [VINP_APSStaSys_enum]
  VVMC_APSActive_flg/1 -> [VVMC_APSActive_flg]

== system vmc/VMC/VMC/APS function/Hand Shake ==
  task_time_s : Inport
  VTQD_ExternalTqAllow_flg : Inport  Port=2
  VTQD_ExtShiftAllow_flg : Inport  Port=3
  VINP_APSVMCReqA_flg : Inport  Port=4
  VINP_APSStaSys_enum : Inport  Port=5
  VTQD_ExtDoorAllow_flg : Inport  Port=6
  AND : Logic  Inputs=3  AllPortsSameDT=off  OutDataTypeStr=boolean
  AND1 : Logic  Inputs=3  AllPortsSameDT=off  OutDataTypeStr=boolean
  AND2 : Logic  AllPortsSameDT=off  OutDataTypeStr=boolean
  Constant : Constant  Value=KVMC_ExternalTqAllowTime_s
  Constant1 : Constant  Value=KVMC_ExternalShiftAllowTime_s
  Constant2 : Constant  Value=ENUM_APSSYSTEMSTA_ACTIVE
  Constant3 : Constant  Value=ENUM_APSSYSTEMSTA_REMOTEACTIVE
  Constant4 : Constant  Value=KVMC_ExternalDoorAllowTime_s
  Delay : Delay  DelayLength=1
  Delay1 : Delay  DelayLength=1
  DelayEnable : hcu_lib/Basic_Blocks/DelayEnable
  DelayEnable1 : hcu_lib/Basic_Blocks/DelayEnable
  DelayEnable2 : hcu_lib/Basic_Blocks/DelayEnable
  Detect Decrease : simulink/Logic and Bit Operations/Detect Decrease  vinit=0.0  OutDataTypeStr=boolean
  Equal : RelationalOperator  Operator===  OutDataTypeStr=boolean  RndMeth=Simplest
  Equal1 : RelationalOperator  Operator===  OutDataTypeStr=boolean  RndMeth=Simplest
  NOT : Logic  Operator=NOT  AllPortsSameDT=off  OutDataTypeStr=boolean
  OR : Logic  Operator=OR  AllPortsSameDT=off  OutDataTypeStr=boolean
  SR_Latch : hcu_lib/Basic_Blocks/SR_Latch
  VVMC_APSCtrlAvail_flg : Outport
  VVMC_APSActive_flg : Outport  Port=2
  wires:
  VINP_APSVMCReqA_flg/1 -> [VINP_APSVMCReqA_flg]
  VTQD_ExtShiftAllow_flg/1 -> [VTQD_ExtShiftAllow_flg]
  [task_time_s] -> DelayEnable1/3
  Constant1/1 -> DelayEnable1/2
  DelayEnable1/1 -> [VVMC_APSShiftCtrlAllow_flg]  "VVMC_APSShiftCtrlAllow_flg"
  [VTQD_ExtShiftAllow_flg] -> DelayEnable1/1
  [VTQD_ExternalTqAllow_flg] -> DelayEnable/1
  VTQD_ExternalTqAllow_flg/1 -> [VTQD_ExternalTqAllow_flg]
  task_time_s/1 -> [task_time_s]
  DelayEnable/1 -> [VVMC_APSTqCtrlAllow_flg]  "VVMC_APSTqCtrlAllow_flg"
  Constant/1 -> DelayEnable/2
  [task_time_s] -> DelayEnable/3
  Constant2/1 -> Equal/2
  [VINP_APSStaSys_enum] -> Equal/1
  Equal/1 -> OR/1
  OR/1 -> AND1/3
  [VINP_APSVMCReqA_flg] -> AND1/1
  Constant3/1 -> Equal1/2
  Equal1/1 -> OR/2
  [VINP_APSStaSys_enum] -> Equal1/1
  [VVMC_APSCtrlAvail_flg] -> AND1/2
  AND1/1 -> [VVMC_APSActive_flg], VVMC_APSActive_flg/1  "VVMC_APSActive_flg"
  VINP_APSStaSys_enum/1 -> [VINP_APSStaSys_enum]
  VTQD_ExtDoorAllow_flg/1 -> [VTQD_ExtDoorAllow_flg]
  Constant4/1 -> DelayEnable2/2
  DelayEnable2/1 -> [VVMC_APSDoorCtrlAllow_flg]  "VVMC_APSDoorCtrlAllow_flg"
  [task_time_s] -> DelayEnable2/3
  [VTQD_ExtDoorAllow_flg] -> DelayEnable2/1
  [VVMC_APSActive_flg] -> Delay1/1
  SR_Latch/1 -> AND/3
  [VVMC_APSActive_flg] -> Delay/1
  Delay/1 -> NOT/1
  NOT/1 -> AND2/2
  AND2/1 -> SR_Latch/1
  Delay1/1 -> Detect Decrease/1
  Detect Decrease/1 -> SR_Latch/2
  [VVMC_APSDoorCtrlAllow_flg] -> AND2/1
  AND/1 -> [VVMC_APSCtrlAvail_flg], VVMC_APSCtrlAvail_flg/1  "VVMC_APSCtrlAvail_flg"
  [VVMC_APSTqCtrlAllow_flg] -> AND/1
  [VVMC_APSShiftCtrlAllow_flg] -> AND/2

== system vmc/VMC/VMC/APS function/Signal Rounting1 ==
  VINP_SCPSystemMode_enum : Inport
  VVMC_APSActive_flg : Inport  Port=2
  VVMC_ADASActive_flg : Inport  Port=3
  VTQD_GearActualPosn_enum : Inport  Port=4
  VVMC_CAASActive_flg : Inport  Port=5
  VTQD_APSStaSys_enum : Inport  Port=6
  VTQD_APSDecReqA_flg : Inport  Port=7
  VTQD_APSDecReq_mps2 : Inport  Port=8
  VTQD_APSReq_enum : Inport  Port=9
  VINP_APSStaSystem_enum : Inport  Port=10
  VINP_APSDecReqA_flg : Inport  Port=11
  VINP_APSDecReq_mps2 : Inport  Port=12
  VINP_APSReq_enum : Inport  Port=13
  Signal Determination VINP_APSDecReqAtest_flg : Subsystem
  Signal Determination VINP_APSDecReqtest_mps2 : Subsystem
  Signal Determination VINP_APSReqtest_enum : Subsystem
  Signal Determination VINP_APSStaSystemtest_enum : Subsystem
  VVMC_APSStaSys_enum : Outport
  VVMC_APSDecReqA_flg : Outport  Port=2
  VVMC_APSDecReq_mps2 : Outport  Port=3
  VVMC_APSReq_enum : Outport  Port=4
  wires:
  [VINP_SCPSystemMode_enum] -> Signal Determination VINP_APSDecReqtest_mps2/3(VINP_SCPSystemMode_enum)
  Signal Determination VINP_APSDecReqAtest_flg/1(SignalOutp) -> VVMC_APSDecReqA_flg/1  "VVMC_APSDecReqA_flg"
  Signal Determination VINP_APSReqtest_enum/1(SignalOutp) -> VVMC_APSReq_enum/1  "VVMC_APSReq_enum"
  [VINP_SCPSystemMode_enum] -> Signal Determination VINP_APSReqtest_enum/3(VINP_SCPSystemMode_enum)
  Signal Determination VINP_APSStaSystemtest_enum/1(SignalOutp) -> VVMC_APSStaSys_enum/1  "VVMC_APSStaSys_enum"
  [VINP_SCPSystemMode_enum] -> Signal Determination VINP_APSDecReqAtest_flg/3(VINP_SCPSystemMode_enum)
  Signal Determination VINP_APSDecReqtest_mps2/1(SignalOutp) -> VVMC_APSDecReq_mps2/1  "VVMC_APSDecReq_mps2"
  VINP_SCPSystemMode_enum/1 -> [VINP_SCPSystemMode_enum]
  VVMC_APSActive_flg/1 -> [VVMC_APSActive_flg]
  VVMC_ADASActive_flg/1 -> [VVMC_ADASActive_flg]
  [VVMC_APSActive_flg] -> Signal Determination VINP_APSStaSystemtest_enum/4(VVMC_APSActive_flg)
  [VVMC_ADASActive_flg] -> Signal Determination VINP_APSStaSystemtest_enum/5(VVMC_ADASActive_flg)
  [VVMC_APSActive_flg] -> Signal Determination VINP_APSDecReqAtest_flg/4(VVMC_APSActive_flg)
  [VVMC_ADASActive_flg] -> Signal Determination VINP_APSDecReqAtest_flg/5(VVMC_ADASActive_flg)
  [VVMC_APSActive_flg] -> Signal Determination VINP_APSDecReqtest_mps2/4(VVMC_APSActive_flg)
  [VVMC_ADASActive_flg] -> Signal Determination VINP_APSDecReqtest_mps2/5(VVMC_ADASActive_flg)
  [VVMC_APSActive_flg] -> Signal Determination VINP_APSReqtest_enum/4(VVMC_APSActive_flg)
  [VVMC_ADASActive_flg] -> Signal Determination VINP_APSReqtest_enum/5(VVMC_ADASActive_flg)
  VTQD_GearActualPosn_enum/1 -> [VTQD_GearActualPosn_enum]
  [VTQD_GearActualPosn_enum] -> Signal Determination VINP_APSStaSystemtest_enum/6(VTQD_GearActualPosn_enum)
  [VINP_SCPSystemMode_enum] -> Signal Determination VINP_APSStaSystemtest_enum/3(VINP_SCPSystemMode_enum)
  [VINP_APSReq_enum] -> Signal Determination VINP_APSReqtest_enum/1(SignalInput1)
  VVMC_CAASActive_flg/1 -> [VVMC_CAASActive_flg]
  [VVMC_CAASActive_flg] -> Signal Determination VINP_APSStaSystemtest_enum/7(VVMC_CAASActive_flg)
  [VVMC_CAASActive_flg] -> Signal Determination VINP_APSDecReqAtest_flg/6(VVMC_CAASActive_flg)
  [VVMC_CAASActive_flg] -> Signal Determination VINP_APSDecReqtest_mps2/6(VVMC_CAASActive_flg)
  [VVMC_CAASActive_flg] -> Signal Determination VINP_APSReqtest_enum/6(VVMC_CAASActive_flg)
  VTQD_APSDecReq_mps2/1 -> [VTQD_APSDecReq_mps2]
  VTQD_APSReq_enum/1 -> [VTQD_APSReq_enum]
  VTQD_APSDecReqA_flg/1 -> [VTQD_APSDecReqA_flg]
  VTQD_APSStaSys_enum/1 -> [VTQD_APSStaSys_enum]
  [VTQD_APSStaSys_enum] -> Signal Determination VINP_APSStaSystemtest_enum/2(SignalInput2)
  [VTQD_APSDecReqA_flg] -> Signal Determination VINP_APSDecReqAtest_flg/2(SignalInput2)
  [VTQD_APSDecReq_mps2] -> Signal Determination VINP_APSDecReqtest_mps2/2(SignalInput2)
  [VTQD_APSReq_enum] -> Signal Determination VINP_APSReqtest_enum/2(SignalInput2)
  VINP_APSStaSystem_enum/1 -> [VINP_APSStaSystem_enum]
  VINP_APSDecReqA_flg/1 -> [VINP_APSDecReqA_flg]
  VINP_APSReq_enum/1 -> [VINP_APSReq_enum]
  VINP_APSDecReq_mps2/1 -> [VINP_APSDecReq_mps2]
  [VINP_APSDecReq_mps2] -> Signal Determination VINP_APSDecReqtest_mps2/1(SignalInput1)
  [VINP_APSDecReqA_flg] -> Signal Determination VINP_APSDecReqAtest_flg/1(SignalInput1)
  [VINP_APSStaSystem_enum] -> Signal Determination VINP_APSStaSystemtest_enum/1(SignalInput1)

== system vmc/VMC/VMC/CruiseControlFunction/CCActiveDetermination ==
  VTQD_SpdCtrlMode_enum : Inport
  VVMC_FeatArbitrFinal_enum : Inport  Port=2
  VTQD_ExternalTqAllow_flg : Inport  Port=3
  VTQD_SWCSetdownSta_flg : Inport  Port=4
  VTQD_SWCResUpSta_flg : Inport  Port=5
  VINP_VehSpeed_kph : Inport  Port=6
  VVMC_FeatSetSpdForCalcu_kph : Inport  Port=7
  VINP_BrakeSWGPIO_flg : Inport  Port=8
  VTQD_SWCCANCELSta_flg : Inport  Port=9
  VINP_BrkSwSta_flg : Inport  Port=10
  VINP_ADASAEBSta_enum : Inport  Port=11
  VVMC_CCPedalOvrd_flg : Inport  Port=12
  VTQD_GearActualPosn_enum : Inport  Port=13
  VINP_Distanceunit_flg : Inport  Port=14
  " 1" : Constant  Value=KTQD_CCActiveMetSpdLo_kph
  " 2" : Constant  Value=KTQD_CCActiveMetSpdLoMPH_mph
  3 : Constant  Value=KTQD_CCActiveMetSpdHi_kph
  5 : Constant  Value=KTQD_CCActiveMetSpdHiMPH_mph
  AND : Logic  AllPortsSameDT=off  OutDataTypeStr=boolean
  Cast To Single : DataTypeConversion  OutDataTypeStr=uint8
  Cast To Single1 : DataTypeConversion  OutDataTypeStr=boolean
  Cast To Single2 : DataTypeConversion  OutDataTypeStr=boolean
  Cast To Single3 : DataTypeConversion  OutDataTypeStr=single
  Cast To Single4 : DataTypeConversion  OutDataTypeStr=single
  Chart : Stateflow chart  TreatAsAtomicUnit=on
  Constant2 : Constant  Value=KVMC_CCMSASpdWar_kph
  Constant3 : Constant  Value=ENUM_FEATARBITRSTA_CC
  Constant4 : Constant  Value=TRUE
  Constant5 : Constant  Value=FALSE
  Constant6 : Constant  Value=ENUM_CCCRLSTA_ACTIVE
  Constant7 : Constant  Value=ENUM_ADASAEBSTA_ACTIVE
  Constant8 : Constant  Value=ENUM_GEARACTUALPOSN_D
  Delay : Delay  DelayLength=1
  Detect Decrease : simulink/Logic and Bit Operations/Detect Decrease  vinit=0.0  OutDataTypeStr=boolean
  Detect Decrease1 : simulink/Logic and Bit Operations/Detect Decrease  vinit=0.0  OutDataTypeStr=boolean
  Detect Decrease2 : simulink/Logic and Bit Operations/Detect Decrease  vinit=0.0  OutDataTypeStr=boolean
  Relational Operator : RelationalOperator  Operator===  OutDataTypeStr=boolean  RndMeth=Simplest
  Relational Operator1 : RelationalOperator  Operator===  OutDataTypeStr=boolean  RndMeth=Simplest
  Switch2 : Switch  Criteria=u2 > Threshold
  Switch3 : Switch  Criteria=u2 > Threshold
  u2 > 0 : Switch  Criteria=u2 > Threshold
  VVMC_CCCtrlSta_enum : Outport
  VVMC_CCSpdWar_flg : Outport  Port=2
  VVMC_CruzActive_flg : Outport  Port=3
  wires:
  Delay/1 -> Chart/15(VVMC_CCPedalOvrd_flg)
  [VVMC_CCPedalOvrd_flg] -> Delay/1
  VVMC_CCPedalOvrd_flg/1 -> [VVMC_CCPedalOvrd_flg]
  Constant7/1 -> Chart/14(ENUM_ADASAEBSTA_ACTIVE)
  [VINP_ADASAEBSta_enum] -> Chart/13(VINP_ADASAEBSta_enum)
  VINP_ADASAEBSta_enum/1 -> [VINP_ADASAEBSta_enum]
  Relational Operator1/1 -> AND/2
  Relational Operator/1 -> AND/1
  [VVMC_CCCtrlSta_enum] -> Relational Operator1/1
  Constant6/1 -> Relational Operator1/2
  Constant5/1 -> u2 > 0/3
  Constant4/1 -> u2 > 0/1
  AND/1 -> u2 > 0/2
  [VTQD_SpdCtrlMode_enum] -> Chart/1(VTQD_SpdCtrlMode_enum)
  VTQD_SpdCtrlMode_enum/1 -> [VTQD_SpdCtrlMode_enum]
  Constant3/1 -> Relational Operator/2
  Switch2/1 -> Cast To Single3/1
  [VINP_VehSpeed_kph] -> Chart/5(VINP_VehSpeed_kph)
  Switch3/1 -> Cast To Single4/1
  [VTQD_SWCSetdownSta_flg] -> Detect Decrease/1
  [VVMC_FeatSetSpdForCalcu_kph] -> Chart/7(VVMC_FeatSetSpdForCalcu_kph)
  Constant2/1 -> Chart/8(KVMC_CCMSASpdWar_kph)
  [VTQD_ExternalTqAllow_flg] -> Chart/2(VTQD_ExternalTqAllow_flg)
  [VVMC_FeatArbitrFinal_enum] -> Relational Operator/1
  [VINP_BrakeSWGPIO_flg] -> Chart/9(VINP_BrakeSWGPIO_flg)
  [VTQD_SWCCANCELSta_flg] -> Detect Decrease1/1
  [VTQD_SWCResUpSta_flg] -> Detect Decrease2/1
  Chart/1(VVMC_CCCtrlSta_enum) -> Cast To Single/1
  Chart/2(VVMC_CCSpdWar_flg) -> Cast To Single1/1
  u2 > 0/1 -> Cast To Single2/1
  VVMC_FeatArbitrFinal_enum/1 -> [VVMC_FeatArbitrFinal_enum]
  VTQD_ExternalTqAllow_flg/1 -> [VTQD_ExternalTqAllow_flg]
  VTQD_SWCSetdownSta_flg/1 -> [VTQD_SWCSetdownSta_flg]
  VTQD_SWCResUpSta_flg/1 -> [VTQD_SWCResUpSta_flg]
  VINP_VehSpeed_kph/1 -> [VINP_VehSpeed_kph]
  VVMC_FeatSetSpdForCalcu_kph/1 -> [VVMC_FeatSetSpdForCalcu_kph]
  VINP_BrakeSWGPIO_flg/1 -> [VINP_BrakeSWGPIO_flg]
  VTQD_SWCCANCELSta_flg/1 -> [VTQD_SWCCANCELSta_flg]
  VINP_BrkSwSta_flg/1 -> [VINP_BrkSwSta_flg]
  [VVMC_CCCtrlSta_enum] -> VVMC_CCCtrlSta_enum/1
  [VVMC_CCSpdWar_flg] -> VVMC_CCSpdWar_flg/1
  [VVMC_CruzActive_flg] -> VVMC_CruzActive_flg/1
  Detect Decrease/1 -> Chart/3(VVMC_DetectSWCSetDown_flg)  "VVMC_DetectSWCSetDown_flg"
  Detect Decrease1/1 -> Chart/10(VVMC_DetectSWCCANCEL_flg)  "VVMC_DetectSWCCANCEL_flg"
  Detect Decrease2/1 -> Chart/12(VVMC_DetectSWCResUp_flg)  "VVMC_DetectSWCResUp_flg"
  Cast To Single1/1 -> [VVMC_CCSpdWar_flg]  "VVMC_CCSpdWar_flg"
  Cast To Single2/1 -> [VVMC_CruzActive_flg]  "VVMC_CruzActive_flg"
  Cast To Single/1 -> [VVMC_CCCtrlSta_enum]  "VVMC_CCCtrlSta_enum"
  [VINP_BrkSwSta_flg] -> Chart/11(VINP_BrkSwSta_flg)
  VTQD_GearActualPosn_enum/1 -> [VTQD_GearActualPosn_enum]
  [VTQD_GearActualPosn_enum] -> Chart/16(VTQD_GearActualPosn_enum)
  Constant8/1 -> Chart/17(ENUM_GEARACTUALPOSN_D)
  3/1 -> Switch2/3
  5/1 -> Switch2/1
  [VINP_Distanceunit_flg] -> Switch2/2
  " 2"/1 -> Switch3/1
  [VINP_Distanceunit_flg] -> Switch3/2
  " 1"/1 -> Switch3/3
  VINP_Distanceunit_flg/1 -> [VINP_Distanceunit_flg]
  Cast To Single3/1 -> Chart/4(KVMC_CCActiveMetSpdHi_kph)
  Cast To Single4/1 -> Chart/6(KVMC_CCActiveMetSpdLo_kph)
